simulink model "MatlabNonlinearStateEstimationForActuatorDelay"  (R2020b)
settings: Solver=VariableStepAuto  StartTime=0.0  StopTime=10  RelTol=1e-3
PostLoadFcn:
  | t0 = 0;
values from neighbouring files (symbols this model uses):
  cg = temp(4)    [NonlinearStateEstimationForActuatorDelay.m]
  Croll = Croll_p + .0001 * (rand - 0.5)    [Forces_and_Moments_Calculator.m]
  Cside = 0    [Forces_and_Moments_Calculator.m]
  Cyaw = Cyaw + .1 * (rand - 0.5)    [Forces_and_Moments_Calculator.m]
  F = eye(6)    [MEKFAttitudeOnly.m]
  I = reshape(x(1:9), [3 3])    [AdaptiveLQR.m]    (also in MEKF.m = diag([0.08 0.08 0.002]); MEKFAttitudeOnly.m = diag([0.08 0.08 0.002]); MEKF_old.m = diag([0.08 0.08 0.002]); NonlinearStateEstimationForActuatorDelay.m = diag([Ixx, Ixx, Izz]))
  mass = 1.0565    [ImpactVelocityNotParallelMatlab.m]    (also in NonlinearStateEstimationForActuatorDelay.m = temp(1); OneDLanding.m; RunImpactVelocityParforCompiled.m; Tracker.m = 1.0616753546)
  q = x(13:16)    [AdaptiveLQR.m]    (also in MEKF.m = nominal_state(4:7); MEKFAttitudeOnly.m = [1 0 0 0]; MEKF_old.m = nominal_state(4:7); NonlinearStateEstimationForActuatorDelay.m = x(4:7))
  r = sym('r', [3 1])    [StateSpaceController.m]    (also in TimeDelayCompensationElevator.m = [0;0]; Tracker.m = [0; 0; -(rocket_length - Average_cg)])
  ThrustTable = xlsread('F15_Thrust','Sheet1')    [ImpactVelocityNotParallelMatlab.m]    (also in OneDLanding.m; ParallelImpactVelocity.m; RunImpactVelocityParforCompiled.m)
undefined symbols (not defined in the file or in its folder): Earth, HeightAboveSeaLevel, Light, masscgI, MIL, WGS84
libraries: shared6dof x5, simulink x3, aerolibwind2 x3, vrlib x2, sharedutil x2, aerolibasang x2, shared6dofsys x2, sharedtransform x2, aerolibatmos2 x1, aerolibbdyn x1, aerolibconvert2 x1, aerolibtransform2 x1
(part 2 of 2)

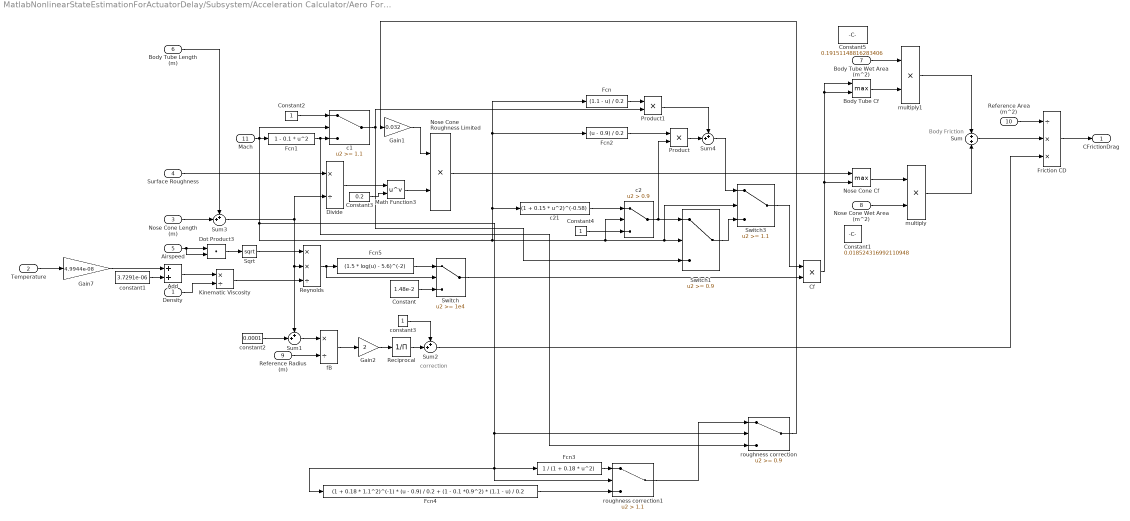
== system MatlabNonlinearStateEstimationForActuatorDelay/Subsystem/Acceleration Calculator/Aero Forces and Moments/Axial Drag Calculator/Friction Drag Calculator ==
  note: correction
  note: Body Friction
  Density : Inport
  Temperature : Inport  Port=2
  Nose Cone Length (m) : Inport  Port=3
  Surface Roughness : Inport  Port=4
  Airspeed : Inport  Port=5
  Body Tube Length (m) : Inport  Port=6
  Body Tube Wet Area (m^2) : Inport  Port=7
  Nose Cone Wet Area (m^2) : Inport  Port=8
  Reference Radius (m) : Inport  Port=9
  Reference Area (m^2) : Inport  Port=10
  Mach : Inport  Port=11
  Add : Sum
  Body Tube Cf : MinMax  Function=max  Inputs=2
  Cf : Product  Inputs=**
  Constant : Constant  Value=1.48e-2
  Constant1 : Constant  Value=0.018524316992110948
  Constant2 : Constant
  Constant3 : Constant  Value=0.2
  Constant4 : Constant
  Constant5 : Constant  Value=0.19151148816283406
  Divide : Product  Inputs=*/
  Dot Product3 : DotProduct  SaturateOnIntegerOverflow=on  OutDataTypeStr=Inherit: Inherit via internal rule
  Fcn : Fcn  Expr=(1.1 - u) / 0.2
  Fcn1 : Fcn  Expr=1 - 0.1 * u^2
  Fcn2 : Fcn  Expr=(u - 0.9) / 0.2
  Fcn3 : Fcn  Expr=1 / (1 + 0.18 * u^2)
  Fcn4 : Fcn  Expr=(1 + 0.18 * 1.1^2)^(-1) * (u - 0.9) / 0.2 + (1 - 0.1 *0.9^2) * (1.1 - u) / 0.2
  Fcn5 : Fcn  Expr=(1.5 * log(u) - 5.6)^(-2)
  Friction CD : Product  Inputs=/**
  Gain1 : Gain  Gain=0.032
  Gain2 : Gain  Gain=2
  Gain7 : Gain  Gain=4.9944e-08
  Kinematic Viscosity : Product  Inputs=*/
  Math Function3 : Math  Operator=pow  SignedPower=on  SaturateOnIntegerOverflow=on
  Nose Cone Cf : MinMax  Function=max  Inputs=2
  Nose Cone Roughness Limited : Product  Inputs=**
  Product : Product
  Product1 : Product
  Reciprocal : Product  Inputs=/
  Reynolds : Product  Inputs=**/
  Sqrt : Sqrt  SaturateOnIntegerOverflow=on
  Sum : Sum
  Sum{1..4} (4 alike) : Sum  Inputs=++|
  Switch : Switch  Threshold=1e4
  Switch1 : Switch  Threshold=0.9
  Switch3 : Switch  Threshold=1.1
  c1 : Switch  Threshold=1.1
  c2 : Switch  Criteria=u2 > Threshold  Threshold=0.9
  c21 : Fcn  Expr=(1 + 0.15 * u^2)^(-0.58)
  constant1 : Constant  Value=3.7291e-06
  constant2 : Constant  Value=0.0001
  constant3 : Constant
  fB : Product  Inputs=*/
  multiply : Product  Inputs=**
  multiply1 : Product  Inputs=**
  roughness correction : Switch  Threshold=0.9
  roughness correction1 : Switch  Criteria=u2 > Threshold  Threshold=1.1
  CFrictionDrag : Outport  VectorParamsAs1DForOutWhenUnconnected=off
  wires:
  Sqrt/1 -> Reynolds/1
  Kinematic Viscosity/1 -> Reynolds/3
  Constant3/1 -> Math Function3/2
  constant1/1 -> Add/2
  Add/1 -> Kinematic Viscosity/1
  Gain7/1 -> Add/1
  Reynolds/1 -> Switch/2, Fcn5/1
  Gain1/1 -> Nose Cone Roughness Limited/1
  Divide/1 -> Math Function3/1
  Math Function3/1 -> Nose Cone Roughness Limited/2
  Surface Roughness/1 -> Divide/1
  Temperature/1 -> Gain7/1
  Density/1 -> Kinematic Viscosity/2
  Nose Cone Roughness Limited/1 -> Nose Cone Cf/1
  Nose Cone Length (m)/1 -> Sum3/2
  Body Tube Length (m)/1 -> Sum3/1
  Cf/1 -> Body Tube Cf/1, Body Tube Cf/2, Nose Cone Cf/2
  Nose Cone Cf/1 -> multiply/1
  Nose Cone Wet Area (m^2)/1 -> multiply/2
  Body Tube Wet Area (m^2)/1 -> multiply1/1
  Body Tube Cf/1 -> multiply1/2
  multiply/1 -> Sum/2
  multiply1/1 -> Sum/1
  constant2/1 -> Sum1/2
  Sum1/1 -> fB/1
  Reference Radius (m)/1 -> fB/2
  fB/1 -> Gain2/1
  Gain2/1 -> Reciprocal/1
  Reciprocal/1 -> Sum2/2
  constant3/1 -> Sum2/1
  Sum/1 -> Friction CD/2
  Sum2/1 -> Friction CD/3
  Reference Area (m^2)/1 -> Friction CD/1
  Friction CD/1 -> CFrictionDrag/1
  Airspeed/1 -> Dot Product3/2, Dot Product3/1
  Dot Product3/1 -> Sqrt/1
  Switch/1 -> Cf/2
  Fcn5/1 -> Switch/1
  Constant/1 -> Switch/3
  c1/1 -> Product1/2, Switch1/3
  Fcn1/1 -> roughness correction/3, c1/3
  Constant2/1 -> c1/1
  c2/1 -> Product/2, Switch1/1
  Constant4/1 -> c2/3
  c21/1 -> c2/1
  Switch3/1 -> Cf/1
  Switch1/1 -> Switch3/3
  Fcn2/1 -> Product/1
  Product/1 -> Sum4/2
  Product1/1 -> Sum4/1
  Fcn/1 -> Product1/1
  Sum4/1 -> Switch3/1
  Fcn3/1 -> roughness correction1/1
  Mach/1 -> roughness correction/2, Fcn4/1, roughness correction1/2, Fcn3/1, Fcn/1, Fcn2/1, c21/1, c2/2, Switch3/2, Switch1/2, c1/2, Fcn1/1
  Fcn4/1 -> roughness correction1/3
  roughness correction1/1 -> roughness correction/1
  roughness correction/1 -> Gain1/1
  Sum3/1 -> Divide/2, Sum1/1, Reynolds/2

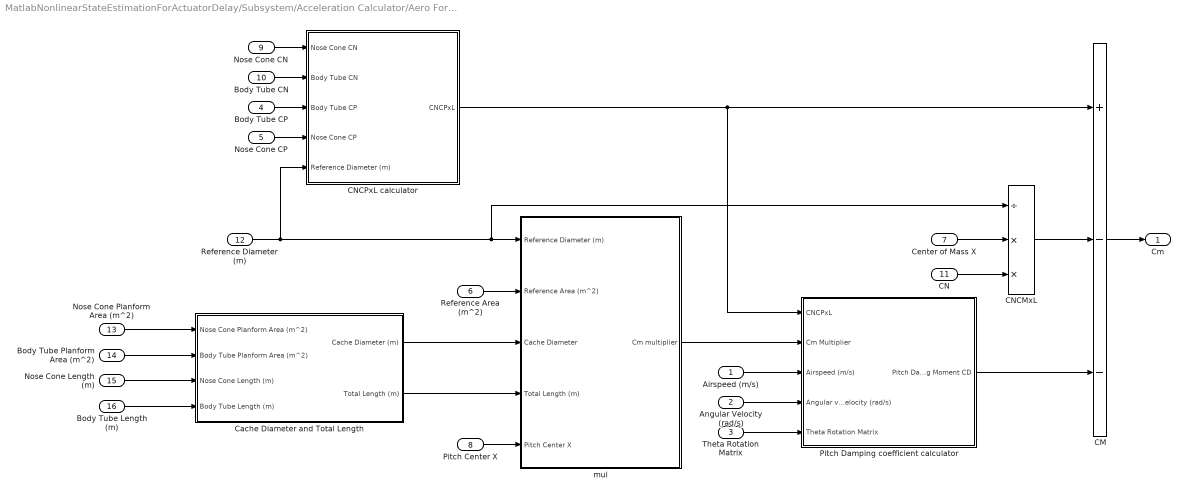
== system MatlabNonlinearStateEstimationForActuatorDelay/Subsystem/Acceleration Calculator/Aero Forces and Moments/CN and Cm calculator/CM calculator ==
  Airspeed (m/s) : Inport
  Angular Velocity (rad/s) : Inport  Port=2
  Theta Rotation Matrix : Inport  Port=3
  Body Tube CP : Inport  Port=4
  Nose Cone CP : Inport  Port=5
  Reference Area (m^2) : Inport  Port=6
  Center of Mass X : Inport  Port=7
  Pitch Center X : Inport  Port=8
  Nose Cone CN : Inport  Port=9
  Body Tube CN : Inport  Port=10
  CN : Inport  Port=11
  Reference Diameter (m) : Inport  Port=12
  Nose Cone Planform Area (m^2) : Inport  Port=13
  Body Tube Planform Area (m^2) : Inport  Port=14
  Nose Cone Length (m) : Inport  Port=15
  Body Tube Length (m) : Inport  Port=16
  CM : Sum  Inputs=+--
  CNCMxL : Product  Inputs=/**
  CNCPxL calculator : Subsystem
  Cache Diameter and Total Length : Subsystem
  Pitch Damping coefficient calculator : Subsystem
  mul : Subsystem
  Cm : Outport  VectorParamsAs1DForOutWhenUnconnected=off
  wires:
  CNCPxL calculator/1("CNCPxL ") -> Pitch Damping coefficient calculator/1(CNCPxL), CM/1
  Pitch Center X/1 -> mul/5(Pitch Center X)
  Cache Diameter and Total Length/2(Total Length (m)) -> mul/4(Total Length (m))
  Reference Diameter (m)/1 -> CNCMxL/1, mul/1(Reference Diameter (m)), CNCPxL calculator/5(Reference Diameter (m))
  Nose Cone CP/1 -> CNCPxL calculator/4(Nose Cone CP)
  CM/1 -> Cm/1
  Body Tube CP/1 -> CNCPxL calculator/3(Body Tube CP)
  Cache Diameter and Total Length/1(Cache Diameter (m)) -> mul/3(Cache Diameter)
  mul/1(Cm multiplier) -> Pitch Damping coefficient calculator/2(Cm Multiplier)
  Angular Velocity (rad/s)/1 -> Pitch Damping coefficient calculator/4(Angular velocity (rad/s))
  Airspeed (m/s)/1 -> Pitch Damping coefficient calculator/3(Airspeed (m/s))
  Reference Area (m^2)/1 -> mul/2(Reference Area (m^2))
  Theta Rotation Matrix/1 -> Pitch Damping coefficient calculator/5(Theta Rotation Matrix)
  Body Tube CN/1 -> CNCPxL calculator/2(Body Tube CN)
  Nose Cone CN/1 -> CNCPxL calculator/1(Nose Cone CN)
  Nose Cone Planform Area (m^2)/1 -> Cache Diameter and Total Length/1(Nose Cone Planform Area (m^2))
  Body Tube Planform Area (m^2)/1 -> Cache Diameter and Total Length/2(Body Tube Planform Area (m^2))
  Nose Cone Length (m)/1 -> Cache Diameter and Total Length/3(Nose Cone Length (m))
  Body Tube Length (m)/1 -> Cache Diameter and Total Length/4(Body Tube Length (m))
  Center of Mass X/1 -> CNCMxL/2
  CN/1 -> CNCMxL/3
  Pitch Damping coefficient calculator/1(Pitch Damping Moment CD) -> CM/3
  CNCMxL/1 -> CM/2

== system MatlabNonlinearStateEstimationForActuatorDelay/Subsystem/Acceleration Calculator/Aero Forces and Moments/CN and Cm calculator/CN calculator ==
  Reference Area (m^2) : Inport
  AoA (rads) : Inport  Port=2
  Mach : Inport  Port=3
  Nose Cone Planform Area (m^2) : Inport  Port=4
  Body Tube Planform Area (m^2) : Inport  Port=5
  CN multiplier : Subsystem
  Component CN : Subsystem
  Normal Force CD : Sum
  Nose Cone CN : Outport  VectorParamsAs1DForOutWhenUnconnected=off
  Body Tube CN : Outport  Port=2  VectorParamsAs1DForOutWhenUnconnected=off
  CN : Outport  Port=3  VectorParamsAs1DForOutWhenUnconnected=off
  wires:
  Mach/1 -> CN multiplier/2(Mach)
  CN multiplier/1(CN multiplier) -> Component CN/2(CN multiplier)
  Component CN/1(Nose Cone CN) -> Normal Force CD/1, Nose Cone CN/1
  AoA (rads)/1 -> CN multiplier/1(AoA (rads)), Component CN/1(AoA (rads))
  Nose Cone Planform Area (m^2)/1 -> Component CN/4(Nose Cone Planform Area)
  Component CN/2(Body Tube CN) -> Normal Force CD/2, Body Tube CN/1
  Body Tube Planform Area (m^2)/1 -> Component CN/5(Body Tube Planform Area)
  Reference Area (m^2)/1 -> Component CN/3(Reference Area)
  Normal Force CD/1 -> CN/1

== system MatlabNonlinearStateEstimationForActuatorDelay/Subsystem/Acceleration Calculator/Aero Forces and Moments/CN and Cm calculator/CM calculator/CNCPxL calculator ==
  Nose Cone CN : Inport
  Body Tube CN : Inport  Port=2
  Body Tube CP : Inport  Port=3
  Nose Cone CP : Inport  Port=4
  Reference Diameter (m) : Inport  Port=5
  Add1 : Sum
  CNCPxL : Product  Inputs=*/
  CNCPxL1 : Product  Inputs=*/
  CNCPxL2 : Product  Inputs=*/
  Product1 : Product
  Product3 : Product
  "CNCPxL " : Outport  VectorParamsAs1DForOutWhenUnconnected=off
  wires:
  Product1/1 -> Add1/1, CNCPxL2/1
  CNCPxL/1 -> "CNCPxL "/1
  Nose Cone CN/1 -> Product1/1
  Reference Diameter (m)/1 -> CNCPxL2/2, CNCPxL1/2, CNCPxL/2
  Body Tube CN/1 -> Product3/1
  Add1/1 -> CNCPxL/1
  Body Tube CP/1 -> Product3/2
  Product3/1 -> CNCPxL1/1, Add1/2
  Nose Cone CP/1 -> Product1/2

== system MatlabNonlinearStateEstimationForActuatorDelay/Subsystem/Acceleration Calculator/Aero Forces and Moments/CN and Cm calculator/CM calculator/Cache Diameter and Total Length ==
  Nose Cone Planform Area (m^2) : Inport
  Body Tube Planform Area (m^2) : Inport  Port=2
  Nose Cone Length (m) : Inport  Port=3
  Body Tube Length (m) : Inport  Port=4
  Cache Diameter : Product  Inputs=*/
  Total Length : Sum
  Total Planform Area : Sum
  Cache Diameter (m) : Outport  VectorParamsAs1DForOutWhenUnconnected=off
  Total Length (m) : Outport  Port=2  VectorParamsAs1DForOutWhenUnconnected=off
  wires:
  Total Planform Area/1 -> Cache Diameter/1
  Nose Cone Planform Area (m^2)/1 -> Total Planform Area/1
  Body Tube Length (m)/1 -> Total Length/2
  Nose Cone Length (m)/1 -> Total Length/1
  Body Tube Planform Area (m^2)/1 -> Total Planform Area/2
  Total Length/1 -> Total Length (m)/1, Cache Diameter/2
  Cache Diameter/1 -> Cache Diameter (m)/1

== system MatlabNonlinearStateEstimationForActuatorDelay/Subsystem/Acceleration Calculator/Aero Forces and Moments/CN and Cm calculator/CM calculator/Pitch Damping coefficient calculator ==
  CNCPxL : Inport
  Cm Multiplier : Inport  Port=2
  Airspeed (m/s) : Inport  Port=3
  Angular velocity (rad/s) : Inport  Port=4
  Theta Rotation Matrix : Inport  Port=5
  Dot Product3 : DotProduct  SaturateOnIntegerOverflow=on  OutDataTypeStr=Inherit: Inherit via internal rule
  Math Function6 : Math  Operator=square  SignedPower=on  SaturateOnIntegerOverflow=on
  MinMax : MinMax  Inputs=2
  Multiply : Product  Inputs=**/
  Pitch DampingMoment CD : Product
  Pitch Rate : Product  Inputs=*/  Multiplication=Matrix(*)
  Sel6 : Selector  InputPortWidth=3  IndexOptions=Index vector (dialog)  Indices=2  OutputSizes=1
  Sign : Signum
  Pitch Damping Moment CD : Outport  VectorParamsAs1DForOutWhenUnconnected=off
  wires:
  Dot Product3/1 -> Multiply/3
  Airspeed (m/s)/1 -> Dot Product3/2, Dot Product3/1
  Sign/1 -> Pitch DampingMoment CD/1
  CNCPxL/1 -> MinMax/1
  Math Function6/1 -> Multiply/2
  Multiply/1 -> MinMax/2
  Pitch DampingMoment CD/1 -> Pitch Damping Moment CD/1
  Sel6/1 -> Sign/1, Math Function6/1
  MinMax/1 -> Pitch DampingMoment CD/2
  Theta Rotation Matrix/1 -> Pitch Rate/2
  Cm Multiplier/1 -> Multiply/1
  Pitch Rate/1 -> Sel6/1
  Angular velocity (rad/s)/1 -> Pitch Rate/1

== system MatlabNonlinearStateEstimationForActuatorDelay/Subsystem/Acceleration Calculator/Aero Forces and Moments/CN and Cm calculator/CM calculator/mul ==
  Reference Diameter (m) : Inport
  Reference Area (m^2) : Inport  Port=2
  Cache Diameter : Inport  Port=3
  Total Length (m) : Inport  Port=4
  Pitch Center X : Inport  Port=5
  Add : Sum
  Add2 : Sum  Inputs=+-
  Constant2 : Constant  Value=4
  Gain2 : Gain  Gain=3 * 0.275
  Math Function : Math  Operator=pow  SignedPower=on  SaturateOnIntegerOverflow=on
  Math Function1 : Math  Operator=pow  SignedPower=on  SaturateOnIntegerOverflow=on
  Multiply : Product  Inputs=**//
  Cm multiplier : Outport  VectorParamsAs1DForOutWhenUnconnected=off
  wires:
  Math Function1/1 -> Add/2
  Pitch Center X/1 -> Add2/2, Math Function1/1
  Constant2/1 -> Math Function/2, Math Function1/2
  Add/1 -> Multiply/1
  Math Function/1 -> Add/1
  Reference Area (m^2)/1 -> Multiply/4
  Multiply/1 -> Gain2/1
  Add2/1 -> Math Function/1
  Reference Diameter (m)/1 -> Multiply/3
  Gain2/1 -> Cm multiplier/1
  Total Length (m)/1 -> Add2/1
  Cache Diameter/1 -> Multiply/2

== system MatlabNonlinearStateEstimationForActuatorDelay/Subsystem/Acceleration Calculator/Aero Forces and Moments/CN and Cm calculator/CN calculator/CN multiplier ==
  AoA (rads) : Inport
  Mach : Inport  Port=2
  1 : Constant
  Compare To Constant : simulink/Logic and Bit Operations/Compare To Constant  relop=<  const=.05  OutDataTypeStr=boolean
  Compare To Constant1 : simulink/Logic and Bit Operations/Compare To Constant  relop=>  const=pi/4  OutDataTypeStr=boolean
  Gain : Gain  Gain=1/0.05
  Logical Operator : Logic  AllPortsSameDT=off  OutDataTypeStr=boolean
  Square : Math  Operator=square  SignedPower=on  SaturateOnIntegerOverflow=on
  cnmul : Switch  Criteria=u2 > Threshold
  CN multiplier : Outport  VectorParamsAs1DForOutWhenUnconnected=off
  wires:
  AoA (rads)/1 -> Compare To Constant1/1
  Logical Operator/1 -> cnmul/2
  Compare To Constant/1 -> Logical Operator/2
  Mach/1 -> Compare To Constant/1, Gain/1
  Compare To Constant1/1 -> Logical Operator/1
  Square/1 -> cnmul/1
  1/1 -> cnmul/3
  Gain/1 -> Square/1
  cnmul/1 -> CN multiplier/1

== system MatlabNonlinearStateEstimationForActuatorDelay/Subsystem/Acceleration Calculator/Aero Forces and Moments/CN and Cm calculator/CN calculator/Component CN ==
  AoA (rads) : Inport
  CN multiplier : Inport  Port=2
  Reference Area : Inport  Port=3
  Nose Cone Planform Area : Inport  Port=4
  Body Tube Planform Area : Inport  Port=5
  Add : Sum
  BodyTube CN : Product
  Constant : Constant  Value=2
  Divide2 : Product  Inputs=**/
  Gain1 : Gain  Gain=1.1
  NoseCone CN : Product
  Product1 : Product
  Product2 : Product
  Trigonometric Function : Trigonometry
  Nose Cone CN : Outport  VectorParamsAs1DForOutWhenUnconnected=off
  Body Tube CN : Outport  Port=2  VectorParamsAs1DForOutWhenUnconnected=off
  wires:
  Body Tube Planform Area/1 -> Product1/2
  NoseCone CN/1 -> Nose Cone CN/1
  Constant/1 -> Add/1
  Nose Cone Planform Area/1 -> Product2/1
  Add/1 -> NoseCone CN/2
  BodyTube CN/1 -> Body Tube CN/1
  CN multiplier/1 -> Divide2/2
  AoA (rads)/1 -> Trigonometric Function/1
  Divide2/1 -> Gain1/1
  Reference Area/1 -> Divide2/3
  Gain1/1 -> Product2/2, Product1/1
  Product2/1 -> Add/2
  Trigonometric Function/1 -> Divide2/1, BodyTube CN/2, NoseCone CN/1
  Product1/1 -> BodyTube CN/1

== matlab function MatlabNonlinearStateEstimationForActuatorDelay/Subsystem/Acceleration Calculator/Subsystem/AngleOfAtack1 ==
  settings: updateMethod=DISCRETE
  data: Airspeed input; AoA output
function AoA = AngleOfAttack(Airspeed)
    AoA = acos(Airspeed(3) / norm(Airspeed));
        
    if norm(Airspeed) <= .01
        AoA = 0;
    end
end

== matlab function MatlabNonlinearStateEstimationForActuatorDelay/Subsystem/Acceleration Calculator/Forces And Moments simple model ==
  settings: updateMethod=DISCRETE
  data: Mach input; Airspeed input size=[3 1]; AoA input; Density input; Temperature input; DynamicPressure input; CenterOfMassX input; Thrust input; Forces output; body_angular_velocity input; Roll_Torque input; Xe input; Moments output; Weight input; CFrictionDrag output
function [Forces, Moments, CFrictionDrag]  = forces(Mach, Airspeed, AoA, Density, Temperature, DynamicPressure, CenterOfMassX, Thrust, body_angular_velocity, Roll_Torque, Xe, Weight)
    persistent ThetaRotation
    if isempty(ThetaRotation)
         ThetaRotation = eye(3);
    end
    
    persistent Croll_p
    if isempty(Croll_p)
        Croll_p = 0.03 * (rand - 0.5);
    end
    %% Rocket Shape Constants
    Reference_Diameter = 7.62e-2;
    Reference_Radius = Reference_Diameter / 2;
    Reference_Area = Reference_Radius^2 * pi;
    
    NoseCone_Length = 15e-2;
    BodyTube_Length = 80e-2; 
    NoseCone_WetArea = pi * Reference_Radius * NoseCone_Length;          % pi*r*l 
    BodyTube_WetArea = pi * Reference_Radius * 2 * BodyTube_Length;      % pi*d*l
    NoseCone_PlanformArea = Reference_Diameter * NoseCone_Length / 2;
    BodyTube_PlanformArea = Reference_Diameter * BodyTube_Length;
    
    SurfaceRoughness = 20e-6;
    
    sinphi = Reference_Radius / hypot(Reference_Radius, NoseCone_Length);
    BodyTube_CP = 0.55;
    NoseCone_CP = 0.1;
    PitchCenterX = 0;
   
    
    COT_to_COM = .95 - CenterOfMassX; %get actual value and change over time as solid motor burns
    
    %% General Constants
    K = 1.1;
   
    %% Coefficients
    angularrate_local = ThetaRotation \ body_angular_velocity;
    [CN, Cpitch] = CalculatePitchAndNormalCDs(Mach, K, Reference_Diameter, AoA, Airspeed, angularrate_local(2), NoseCone_Length, BodyTube_Length, Reference_Area, CenterOfMassX, PitchCenterX, NoseCone_PlanformArea, BodyTube_PlanformArea, NoseCone_CP, BodyTube_CP);

    Cbase = .12 + .13*Mach^2;
    CFrictionDrag = CalculateFrictionDrag(Temperature, Density, Reference_Radius, Reference_Area, SurfaceRoughness, NoseCone_Length, BodyTube_Length, Airspeed, Mach, NoseCone_WetArea, BodyTube_WetArea);
    Cpressure = PressureDragForce(sinphi);
    
    Cdrag = Cbase + CFrictionDrag + Cpressure;
    Caxial = AxialDragMul(AoA) * Cdrag;

    Cyaw = 0;
    Cside = 0;
    Croll = 0;
    
     %% Random Noise to pitch and yaw coefficients in the range of +- 5e-4
    %Cpitch = Cpitch + .1 * (rand - 0.5);
    %Cyaw = Cyaw + .1 * (rand - 0.5);
    %Croll = Croll_p + .0001 * (rand - 0.5);
    %% Forces and Moments
    lengtha = norm(Airspeed(1:2));
    
    cosa = Airspeed(1) / lengtha;
    sina = Airspeed(2) / lengtha;

    ThetaRotation = [cosa, -sina, 0; sina, cosa, 0; 0, 0, 1];
    
    z = DynamicPressure * Reference_Area;
    Thrust_moment = COT_to_COM * [Thrust(1:2); 0] + [0;0; Roll_Torque];
    
    Forces = ThetaRotation * z * -[CN; Cside; Caxial] + Thrust - Weight;
    Moments = ThetaRotation * (z * Reference_Diameter * [-Cyaw; Cpitch; Croll]) + Thrust_moment;
    
    if Xe(3) <= 0
        Forces = [0;0; dot(Forces, [0,0,1])];
        Moments = [0; 0; 0];
    end
    
end

== matlab function MatlabNonlinearStateEstimationForActuatorDelay/Subsystem2/MATLAB Function1 ==
  settings: updateMethod=DISCRETE
  data: state input; K_x_xy_out output; K_x_roll_out output; time input; k_0_out output; current_u input
function [K_x_xy_out, K_x_roll_out, k_0_out] = fcn(state, time, current_u)
  coder.extrinsic('affine_controller'); 
  persistent last_time K_x k_0

  if isempty(last_time)
    last_time = 0;
    K_x = zeros(3, 9);
    k_0 = zeros(3, 1);
    [K_x, k_0, ~] = affine_controller(state, current_u);
  end
  
  if time - last_time > 10
    [K_x, k_0, ~] = affine_controller(state, current_u);
  end
  
  K_x_xy_out = K_x(1:2, :);
  K_x_roll_out = K_x(3, :);
  k_0_out = k_0;
  
  last_time = time;
  
%   K_x_out = zeros(3, 9);
%   k_0_out = zeros(3, 1);
%   [K_x_out, k_0_out, ~] = affine_controller(state, current_u);
end

== matlab function MatlabNonlinearStateEstimationForActuatorDelay/MATLAB Function2 ==
  settings: updateMethod=DISCRETE
  data: state input; u input; estimatedRollState output; ThrustTable input; time input; masscgI input; estimatedPitchState output
function [estimatedRollState, estimatedPitchState] = fcn(state, u, ThrustTable, time, masscgI)
  coder.extrinsic('NonlinearStateEstimationForActuatorDelay'); 
  persistent all_u
  
  if isempty(all_u)
    all_u = [-10000 0 0 0; -1e-5 0 0 0];
  end
  
  all_u = [all_u; time u'];
  
  estimatedRollState = zeros(15, 1);
  estimatedPitchState = zeros(15, 1);
  [estimatedRollState, estimatedPitchState] = NonlinearStateEstimationForActuatorDelay(state, all_u, ThrustTable, time, [0.07 0.07 0.01], masscgI);
end
